simulink model "asyncip_sl_2_sc_console"  (Simulink 7.8)
settings: Solver=ode4  SolverMode=SingleTasking  StartTime=0.0  StopTime=inf  FixedStep=5e-005  MaxStep=0.01  RelTol=1e-3  AbsTol=1e-6
libraries: opal_lib x1
settings Model: Creator=jwu  LastModifiedBy=ACS  ExtModeTrigMode=oneshot  ExtModeArmWhenConnect=off  BufferReuse=off
settings DataIOCC: ExternalInput=[]  InitialState=[]  LimitDataPoints=off  SaveOutput=off  SaveTime=off  SignalLoggingName=sigsOut
settings OptimizationCC: BooleanDataType=off  OptimizeBlockIOStorage=off  BufferReuse=off  ExpressionFolding=off  FoldNonRolledExpr=off  LocalBlockOutputs=off  InitFltsAndDblsToZero=on
settings DebuggingCC: SaveWithParameterizedLinksMsg=none  SignalResolutionControl=TryResolveAllWithWarning  SolverPrmCheckMsg=none  InheritedTsInSrcMsg=none  MultiTaskDSMMsg=warning  MultiTaskCondExecSysMsg=none  FcnCallInpInsideContextMsg=Use local settings  StrictBusMsg=None
settings HardwareCC: TargetUnknown=on
settings RTWCC: GenCodeOnly=on  IncludeERTFirstTime=on
settings CodeAppCC: IgnoreCustomStorageClasses=off
settings GRTTargetCC: TargetFcnLib=ansi_tfl_tmw.mat

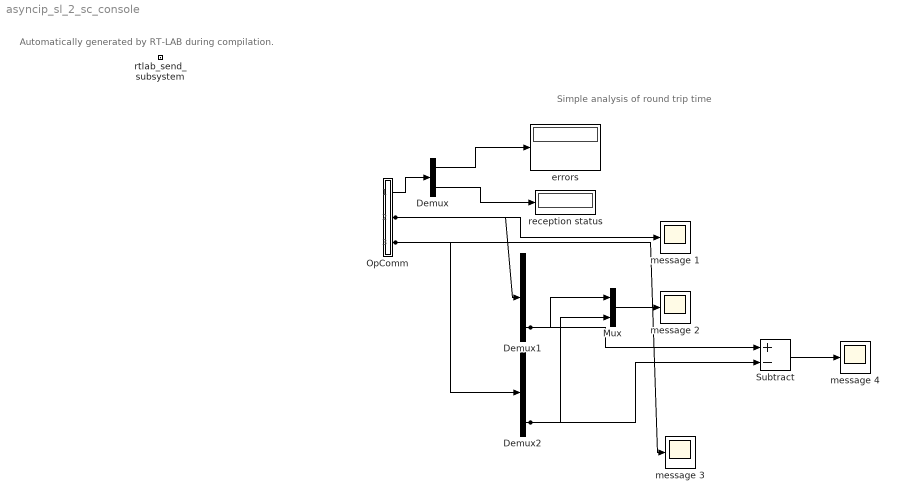
== system asyncip_sl_2_sc_console ==
  note: Simple analysis of round trip time
  note: Automatically generated by RT-LAB during compilation.
  Demux : Demux  Outputs=[2 1]
  Demux1 : Demux  Outputs=5
  Demux2 : Demux  Outputs=5
  Mux : Mux  Inputs=2
  OpComm : Subsystem
      mask init:
      | opmaskdisplay('maskdisplay_block',gcb,'disp(''OpComm'')');
      mask Display:
      | patch([0 0.5 0.7 0],[1 1 0 0],[0.7 0.75 0.9]);
      | patch([1 0.53 0.73 1],[1 1 0 0],[1 0.8 0.7]);
      | plot([0 0 1 1 0],[0 1 1 0 0]);
      | disp('OpComm')
  Subtract : Sum  Inputs=+-
  errors : Display
      settings: Decimation=5000
  message {1..4} (4 alike) : Scope
      message 1 settings: YMin=-1.75  YMax=4
      message 2 settings: YMin=-1.75  YMax=4
      message 3 settings: YMin=-1.75  YMax=4  SaveName=ScopeData2
      message 4 settings: YMin=-1.75  YMax=4  SaveName=ScopeData3
  reception status : Display
      settings: Decimation=5000
  rtlab_send_subsystem : Subsystem  Priority=-100
      mask Display: text(0,0,'');
  wires:
  Demux2/5 -> Mux/2, Subtract/2
  Demux1/5 -> Mux/1, Subtract/1
  Subtract/1 -> message 4/1
  OpComm/3(Out3) -> Demux2/1, message 3/1
  Mux/1 -> message 2/1
  Demux/2 -> reception status/1
  Demux/1 -> errors/1
  OpComm/1(Out1) -> Demux/1
  OpComm/2(Out2) -> Demux1/1, message 1/1

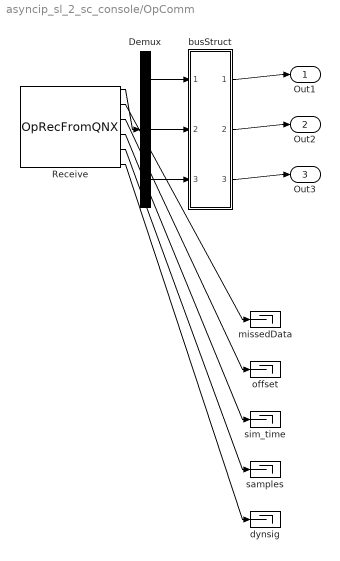
== system asyncip_sl_2_sc_console/OpComm ==
  Demux : Demux  Outputs="[3  5  5]"
  Receive : opal_lib/Communication/OpRecFromQNX  Node_num=1  Acqu_Group=1  Data_Width=13  Synchronization=on  Interpolation=on  Threshold=1.0  modelname=AsyncIP_sl.mdl  sampletime=5e-005
  busStruct : Subsystem
  dynsig : Terminator
  missedData : Terminator
  offset : Terminator
  samples : Terminator
  sim_time : Terminator
  Out1 : Outport
  Out2 : Outport  Port=2
  Out3 : Outport  Port=3
  wires:
  Demux/3 -> busStruct/3(In3)
  Demux/2 -> busStruct/2(In2)
  Demux/1 -> busStruct/1(In1)
  busStruct/3(Out3) -> Out3/1
  busStruct/2(Out2) -> Out2/1
  busStruct/1(Out1) -> Out1/1
  Receive/1 -> Demux/1
  Receive/6 -> dynsig/1
  Receive/5 -> samples/1
  Receive/4 -> sim_time/1
  Receive/3 -> offset/1
  Receive/2 -> missedData/1

== system asyncip_sl_2_sc_console/rtlab_send_subsystem ==

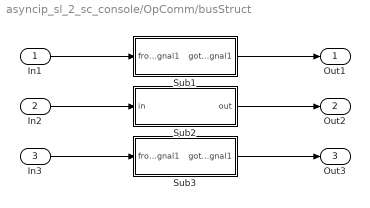
== system asyncip_sl_2_sc_console/OpComm/busStruct ==
  In1 : Inport
  In2 : Inport  Port=2
  In3 : Inport  Port=3
  Sub1 : Subsystem
  Sub2 : Subsystem
  Sub3 : Subsystem
  Out1 : Outport
  Out2 : Outport  Port=2
  Out3 : Outport  Port=3
  wires:
  Sub3/1(goto_signal1) -> Out3/1
  In3/1 -> Sub3/1(from_signal1)
  Sub2/1(out) -> Out2/1
  In2/1 -> Sub2/1(in)
  Sub1/1(goto_signal1) -> Out1/1
  In1/1 -> Sub1/1(from_signal1)

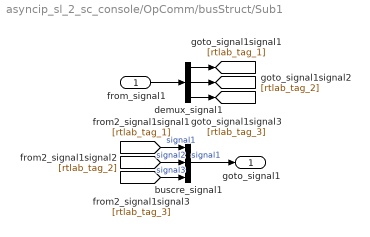
== system asyncip_sl_2_sc_console/OpComm/busStruct/Sub1 ==
  from_signal1 : Inport
  buscre_signal1 : BusCreator  Inputs=3
  demux_signal1 : Demux  Outputs="[1  1  1]"
  goto_signal1 : Outport
  wires:
  buscre_signal1/1 -> goto_signal1/1  "signal1"
  [rtlab_tag_3] -> buscre_signal1/3  "signal3"
  [rtlab_tag_2] -> buscre_signal1/2  "signal2"
  [rtlab_tag_1] -> buscre_signal1/1  "signal1"
  demux_signal1/3 -> [rtlab_tag_3]
  demux_signal1/2 -> [rtlab_tag_2]
  demux_signal1/1 -> [rtlab_tag_1]
  from_signal1/1 -> demux_signal1/1

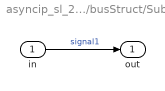
== system asyncip_sl_2_sc_console/OpComm/busStruct/Sub2 ==
  in : Inport
  out : Outport
  wires:
  in/1 -> out/1  "signal1"

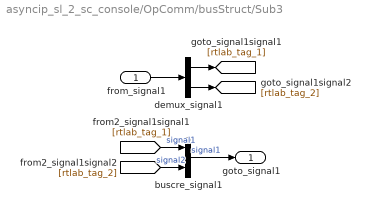
== system asyncip_sl_2_sc_console/OpComm/busStruct/Sub3 ==
  from_signal1 : Inport
  buscre_signal1 : BusCreator  Inputs=2
  demux_signal1 : Demux  Outputs="[4  1]"
  goto_signal1 : Outport
  wires:
  buscre_signal1/1 -> goto_signal1/1  "signal1"
  [rtlab_tag_2] -> buscre_signal1/2  "signal2"
  [rtlab_tag_1] -> buscre_signal1/1  "signal1"
  demux_signal1/2 -> [rtlab_tag_2]
  demux_signal1/1 -> [rtlab_tag_1]
  from_signal1/1 -> demux_signal1/1
